simulink model "mainmodel"  (R2020a)
settings: Solver=VariableStepAuto  StartTime=0.0  StopTime=10.0  RelTol=1e-3
libraries: simulink_extras x1
settings Model: Creator=Bhanu  LastModifiedBy=Bhanu

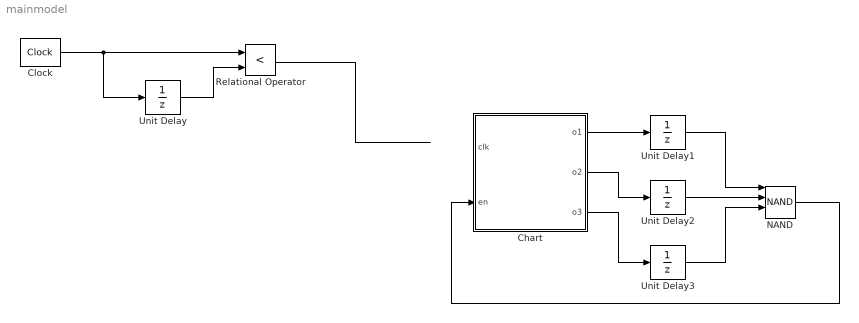
== system mainmodel ==
  Chart : Stateflow chart  TreatAsAtomicUnit=on
  Clock : simulink_extras/Flip Flops/Clock  period=1
  NAND : Logic  Operator=NAND  Inputs=4  IconShape=distinctive  AllPortsSameDT=off  OutDataTypeStr=boolean
  Relational Operator : RelationalOperator  Operator=<  OutDataTypeStr=boolean  RndMeth=Simplest
  Unit Delay{,1..3} (4 alike) : UnitDelay  SampleTime=-1  HasFrameUpgradeWarning=on
  wires:
  Chart/1(o1) -> Unit Delay1/1
  Chart/2(o2) -> Unit Delay2/1
  Chart/3(o3) -> Unit Delay3/1
  NAND/1 -> Chart/2(en)
  Unit Delay1/1 -> NAND/1
  Unit Delay2/1 -> NAND/2
  Unit Delay3/1 -> NAND/3
  Unit Delay/1 -> Relational Operator/2
  Relational Operator/1 -> ?
  Clock/1 -> Relational Operator/1, Unit Delay/1

== stateflow chart mainmodel/Chart ==
  state state1
    en: o1 = 0;
    o2 = 0;
    o3 = 0;
  state state2
    en: o1 = 1;
    o2 = 0;
    o3 = 0;
  state state8
    en: o1 = 1;
    o2 = 1;
    o3 = 1;
  state state3
    en: o1 = 0;
    o2 = 1;
    o3 = 0;
  state state7
    en: o1 = 0;
    o2 = 1;
    o3 = 1;
  state state4
    en: o1 = 1;
    o2 = 1;
    o3 = 0;
  state state5
    en: o1 = 0;
    o2 = 0;
    o3 = 1;
  state state6
    en: o1 = 1;
    o2 = 0;
    o3 = 1;
  (default) -> state1
  state2 -> state3 : [clk == 1]
  state8 -> state1 : [clk == 1]
  state1 -> state2 : [clk == 1]
  (junction 27) -> state1 [order 1] : [en == 1]
  state7 -> state8 : [clk == 1]
  state3 -> state4 : [clk == 1]
  state6 -> state7 : [clk == 1]
  state4 -> state5 : [clk == 1]
  (junction 27) -> state6 [order 2] : [en == 0]
  state5 -> (junction 27) : [clk == 1]
  data: clk input; o1 output; o2 output; o3 output; en input
